simulink model "TRUAV_Dynamics_from_GTRS_trim"  (R2022b)
settings: Solver=ode4  StartTime=0.0  StopTime=3  FixedStep=0.004  RelTol=1e-3
values from neighbouring files (symbols this model uses):
  a_sound = 1116.45    [init_0_GTRS_data_Run_this_file.m]
  alpha_F_rad = alpha_F_deg * (pi/180)    [init_Vetical_2_Table.m]
  alpha_F_rad_table = alpha_F_table * (pi/180)    [init_Fuselage_Aero_Table.m]
  alpha_H_rad = alpha_H_deg * (pi/180)    [init_Horizontal_Table.m]
  alpha_HD_rad = alpha_HD_deg * (pi/180)    [init_Horizontal_C_D_Table.m]
  alpha_r0 = 0    [init_0_GTRS_data_Run_this_file.m]
  alpha_WF_epsilon_M_rad = alpha_WF_deg * pi/180    [init_WingWake_Deflection_Table.m]
  alpha_WS_CL_rad = alpha_WS_CL_deg * (pi/180)    [init_Wing_Slide_Table.m]
  b_w = 32.17    [init_0_GTRS_data_Run_this_file.m]
  beta_F_rad = beta_F_deg * (pi/180)    [init_Vetical_2_Table.m]
  beta_LD_rad_table = beta_LD_table * (pi/180)    [init_Fuselage_Aero_Table.m]
  beta_m_epsilon_M_rad = beta_m_deg * pi/180    [init_WingWake_Deflection_Table.m]
  beta_m_rad_cn = beta_m_deg_cn * pi/180    [init_Wing_Free_Table.m]
  beta_M_rad_table = beta_M_table  * (pi/180)    [init_Fuselage_Aero_Table.m]
  beta_m_S_rad = beta_m_S_deg * (pi/180)    [init_Vetical_2_Table.m]
  beta_m_WS_CL_rad = beta_m_WS_CL_deg * (pi/180)    [init_Wing_Slide_Table.m]
  beta_rad_brk = beta_KBR_rad    [init_Vetical_2_Table.m]
  beta_v_rad = beta_v_deg * (pi/180)    [init_Vetical_1_Table.m]
  beta_vD_rad = beta_vD_deg * (pi/180)    [init_Vetical_1_Table.m]
  beta_WF_Cl_rad = beta_W_deg * (pi/180)    [init_Wing_Free_Table.m]
  beta_WF_CL_rad = beta_CL_deg * (pi/180)    [init_Wing_Free_Table.m]
  beta_YlN_rad_table = beta_YlN_table * (pi/180)    [init_Fuselage_Aero_Table.m]
  c_HW = 3.92    [init_0_GTRS_data_Run_this_file.m]
  C_l_beta_CLwp_table = [ ... (first row only)    [init_Wing_Free_Table.m]
  C_l_beta_pro_CLwp_table = [ ... (first row only)    [init_Wing_Free_Table.m]
  C_L_delta_a_table = [0.00316, 0.00396, 0.00476, 0]    [init_Wing_Free_Table.m]
  C_LHB = -0.00422    [init_0_GTRS_data_Run_this_file.m]
  C_lp_C_LWP = -0.774    [init_0_GTRS_data_Run_this_file.m]
  C_m_wp_table = [ ... (first row only)    [init_Wing_Free_Table.m]
  C_MHA = 0    [init_0_GTRS_data_Run_this_file.m]
  C_MHO = 0    [init_0_GTRS_data_Run_this_file.m]
  c_R = 14/12    (= 1.16666666667)    [init_0_GTRS_data_Run_this_file.m]
  c_w = 5.225    [init_0_GTRS_data_Run_this_file.m]
  C_Y_beta = 0    [init_0_GTRS_data_Run_this_file.m]
  CD0_high_Mach_data = [0.0177, 0.0178, 0.0179, 0.0405]    [init_Wing_Free_Table.m]
  CD_4D_table = zeros(49, 4, 2, 4)    [init_Wing_Slide_Table.m]
  CDH_2D_table = zeros(length(alpha_HD_deg), length(mach_vec))    [init_Horizontal_C_D_Table.m]
  CDV_2D_table = zeros(length(beta_vD_deg), length(mach_vec))    [init_Vetical_1_Table.m]
  CL_4D_table = zeros(49, 4, 2, 4)    [init_Wing_Slide_Table.m]
  CLH_3D_table = zeros(length(alpha_H_deg), length(delta_e_deg), length(mach_vec))    [init_Horizontal_Table.m]
  CYV_3D_table = zeros(length(beta_v_deg), length(delta_r_deg), length(mach_vec))    [init_Vetical_1_Table.m]
  D_alpha_table = [D_part1, D_part2, D_part3, D_part4]    [init_Fuselage_Aero_Table.m]
  D_beta_table = [ fliplr(D_beta_half(2:end)),  D_beta_half]    [init_Fuselage_Aero_Table.m]
  D_ke = 0.24    [init_0_GTRS_data_Run_this_file.m]
  D_Kr = 0.24    [init_0_GTRS_data_Run_this_file.m]    (also in init_Vetical_1_Table.m)
  DBFO = -1.56    [init_0_GTRS_data_Run_this_file.m]
  delta_e_rad = delta_e_deg * (pi/180)    [init_Horizontal_Table.m]
  delta_r_deg = [-20, -15, 0, 15, 20]    [init_Vetical_1_Table.m]
  DLANG = -0.5    [init_0_GTRS_data_Run_this_file.m]
  epsilon_W_table = permute(epsilon_W_3D, [3, 1, 2])    [init_WingWake_Deflection_Table.m]
  flap_rad = flap_deg * (pi/180)    [init_Wing_Free_Table.m]    (also in init_Wing_Slide_Table.m)
  ft2m = 0.3048    [init_0_GTRS_data_Run_this_file.m]
  h_HW = [-0.5838, 0.01158, 0.5967, 0.002547,-2.2519]    [init_0_GTRS_data_Run_this_file.m]
  I_b = 102.5    [init_0_GTRS_data_Run_this_file.m]
  i_H = 0    [init_0_GTRS_data_Run_this_file.m]
  i_v = 0    [init_0_GTRS_data_Run_this_file.m]
  i_w = 0    [init_0_GTRS_data_Run_this_file.m]
  in2ft = 1/12    (= 0.0833333333333)    [init_0_GTRS_data_Run_this_file.m]
  Ixx = 52795    [init_0_GTRS_data_Run_this_file.m]
  Ixz = 1234    [init_0_GTRS_data_Run_this_file.m]
  Iyy = 21360    [init_0_GTRS_data_Run_this_file.m]
  Izz = 66335    [init_0_GTRS_data_Run_this_file.m]
  K1delta_data = [ ... (first row only)    [init_Wing_Free_Table.m]
  K_coeffs = [1.6 0]    [init_0_GTRS_data_Run_this_file.m]
  K_FWDF = -0.0035    [init_0_GTRS_data_Run_this_file.m]
  K_FWO = 1.4    [init_0_GTRS_data_Run_this_file.m]
  K_HNU = 0.8    [init_0_GTRS_data_Run_this_file.m]
  K_vNU = 1    [init_Vetical_1_Table.m]
  KBR_table = KBR_table_full    [init_Vetical_2_Table.m]
  Kn_delta_data = [ ... (first row only)    [init_Wing_Free_Table.m]
  Kno_delta_data = [ ... (first row only)    [init_Wing_Free_Table.m]
  L_alpha_table = [L_part1, L_part2, L_part3, L_part4]    [init_Fuselage_Aero_Table.m]
  L_beta_table = [ fliplr(L_beta_half(2:end)),  L_beta_half]    [init_Fuselage_Aero_Table.m]
  l_beta_table = [l_beta_neg, l_beta_pos]    [init_Fuselage_Aero_Table.m]
  L_n = 4.667    [init_0_GTRS_data_Run_this_file.m]
  lambda_w = -6.5*deg2rad    (= -0.11344640138)    [init_0_GTRS_data_Run_this_file.m]
  LBFO = -7.23    [init_0_GTRS_data_Run_this_file.m]
  LLANG = 0    [init_0_GTRS_data_Run_this_file.m]
  m2ft = 1/ft2m    (= 3.28083989501)    [init_0_GTRS_data_Run_this_file.m]
  M_alpha_table = [M_part1, M_part2, M_part3, M_part4]    [init_Fuselage_Aero_Table.m]
  M_beta_table = [ fliplr(M_beta_half(2:end)), M_beta_half]    [init_Fuselage_Aero_Table.m]
  Mach_brk = [0.2, 0.4, 0.5, 0.6]    [init_Wing_Free_Table.m]
  mach_vec = [0.2, 0.4, 0.5, 0.6]    [init_Horizontal_C_D_Table.m]    (also in init_Horizontal_Table.m; init_Vetical_1_Table.m)
  mass = 403.7    [init_0_GTRS_data_Run_this_file.m]
  mast_rad = mast_deg * pi/180    [init_Wing_Free_Table.m]
  MBFO = 66.5    [init_0_GTRS_data_Run_this_file.m]
  Mn_X_ke = [0 0.2 0.4 0.5 0.6 0.7]    [init_Horizontal_Table.m]
  N_beta_table = [N_beta_neg, N_beta_pos]    [init_Fuselage_Aero_Table.m]
  pos_x_CG = 300    [init_0_GTRS_data_Run_this_file.m]
  pos_x_H = 300    [init_0_GTRS_data_Run_this_file.m]
  pos_x_HW = 560    [init_0_GTRS_data_Run_this_file.m]
  pos_x_Nac = 291.7    [init_0_GTRS_data_Run_this_file.m]
  pos_x_V = 570    [init_0_GTRS_data_Run_this_file.m]
  pos_x_W = 291.7    [init_0_GTRS_data_Run_this_file.m]
  pos_y_CG = 0    [init_0_GTRS_data_Run_this_file.m]
  pos_y_H = 193    [init_0_GTRS_data_Run_this_file.m]
  pos_y_HW = 0    [init_0_GTRS_data_Run_this_file.m]
  pos_y_Nac = 193    [init_0_GTRS_data_Run_this_file.m]
  pos_y_V = 115.69    [init_0_GTRS_data_Run_this_file.m]
  pos_y_W = 96.6    [init_0_GTRS_data_Run_this_file.m]
  pos_z_CG = 81.65    [init_0_GTRS_data_Run_this_file.m]
  pos_z_H = 100    [init_0_GTRS_data_Run_this_file.m]
  pos_z_HW = 103    [init_0_GTRS_data_Run_this_file.m]
  pos_z_Nac = 118    [init_0_GTRS_data_Run_this_file.m]
  pos_z_V = 77    [init_0_GTRS_data_Run_this_file.m]
  pos_z_W = 96    [init_0_GTRS_data_Run_this_file.m]
  R = 12.5    [init_0_GTRS_data_Run_this_file.m]
  rho = 0.002376    [init_0_GTRS_data_Run_this_file.m]
  s_HW = 50.25    [init_0_GTRS_data_Run_this_file.m]
  S_max = 56    [init_0_GTRS_data_Run_this_file.m]
  S_v = 20.25    [init_0_GTRS_data_Run_this_file.m]
  S_w = 181    [init_0_GTRS_data_Run_this_file.m]
  Sidewash_4D = zeros(length(alpha_F_deg), length(beta_F_deg), length(beta_m_S_deg), length(delta_F_S_deg))    [init_Vetical_2_Table.m]
  slugft2kgm = 1.35582    [init_0_GTRS_data_Run_this_file.m]
  tau_e = 0.518    [init_0_GTRS_data_Run_this_file.m]
  tau_r = 0.27    [init_0_GTRS_data_Run_this_file.m]    (also in init_Vetical_1_Table.m)
  theta_0_R = 0.750    (= 0.75)    [init_0_GTRS_data_Run_this_file.m]
  theta_0_W = 1.187    [init_0_GTRS_data_Run_this_file.m]
  theta_twist = -41*deg2rad    (= -0.715584993318)    [init_0_GTRS_data_Run_this_file.m]
  u_max = 1181/12    (= 98.4166666667)    [init_0_GTRS_data_Run_this_file.m]
  ... (+3 more)
undefined symbols (not defined in the file or in its folder): beta_m_rad, F, Light, MIL, sigbuilder_block, tilt_cmd
libraries: simulink x2, sharedtransform x2, aerolibasang x2, aerolibwind2 x1
(part 4 of 4)

== matlab function TRUAV_Dynamics_from_GTRS_trim/Force and Moments/Propulsion1/Rotor Assembly 1 Right/叶素法 ==
  data: para input; AB input; V_H input; r_n input; beta_F_params input; Psi_1 input; v_i input; a_MR input; F_b output; M_b output; delta_H input; T_NAC2B input; T_H2NAC input; beta_F output; Thrust_mag output
function [F_b, M_b, beta_F, Thrust_mag] = F_M_rotor(para,AB, V_H, r_n, beta_F_params, Psi_1, ...
                                           v_i, a_MR, delta_H, T_NAC2B, T_H2NAC)
% =========================================================================
% 全旋翼（3叶片）叶素积分气动力与力矩计算函数
% =========================================================================

    % ========== 0. 参数读取 =============
    R = para(1);
    theta_twist = para(2); % 扭转率
    rho = para(3);
    c_R = para(4);a_sound = para(5);

    Nb = 3;                % 桨叶数 (XV-15/V-22均为3叶)
    
    theta_all = AB(1);     % 总距
    A1 = AB(2); B1 = AB(3); % 横向、纵向周期变距
    
    % 从第二段代码传入的挥舞傅里叶系数
    a0  = beta_F_params(1);
    a1s = beta_F_params(2);
    b1s = beta_F_params(3);

    delta_H = delta_H(:); % 无论输入是什么形状，强行拉直为列向量
    
    N_segments = 40;
    dr = R / N_segments;
    r_vec = (0.5:1:N_segments-0.5)' * dr; 
    x = r_vec / R;
    
    % 初始化整个旋翼在桨毂系(Hub)下的总力和总力矩
    % 初始化整个旋翼在桨毂系(Hub)下的总力和总力矩
    F_HUB_total = zeros(3,1); 
    M_HUB_total = zeros(3,1); 
    
    % ========== 改造点：方位角离散平均法 ==========
    N_azimuth = 36; % 将一圈分为 36 份 (每 10 度算一次)
    dPsi = 2 * pi / N_azimuth;
    
    for k = 1:N_azimuth
        % 虚拟桨叶当前的方位角
        Psi = (k - 1) * dPsi; 
        
        % 根据傅里叶级数实时计算该方位角下的挥舞角和角速度
        beta_F = a0 - a1s*cos(Psi) - b1s*sin(Psi);
        beta_dot = r_n * (a1s*sin(Psi) - b1s*cos(Psi));
        
        dY_prime = zeros(N_segments, 1);
        dZ_prime = zeros(N_segments, 1);
        dQ_torque = zeros(N_segments, 1);
        
        % ========== 2. 逐段计算叶素气动力 ==========
        for i = 1:N_segments
            r_local = r_vec(i);
            
            % 【修复提醒】：请用回正确的面内速度矢量分解！
            % (不要用 sqrt 标量化，否则侧飞时力矩会错)
            U_T = r_n * r_local + V_H(1) * sin(Psi) - V_H(2) * cos(Psi); 
            U_R = V_H(1) * cos(Psi) + V_H(2) * sin(Psi);
            U_P = r_local * beta_dot + U_R * beta_F + V_H(3) + v_i;
            
            if U_T < 0; U_T = abs(U_T); end
            
            phi_b = atan2(U_P, U_T);
            theta = theta_all + A1*cos(Psi) + B1*sin(Psi) + theta_twist*x(i);
            alpha_blade = theta - phi_b;
            
            U = sqrt(U_T^2 + U_P^2);
            M_local = U / a_sound;
            abs_alpha = abs(alpha_blade);
            cd_base = 0.015 + abs_alpha * (0.068 + abs_alpha * 0.81);
            comp_term = 0.01 * abs_alpha + 0.02 *(0.85+ max(M_local,0.35)); 
            cd_comp = max(0, comp_term);
            cd_local = min(0.11, cd_base + cd_comp);
            
            dL = 0.5 * rho * U^2 * a_MR * alpha_blade * c_R * dr;
            dD = 0.5 * rho * U^2 * cd_local * c_R * dr;
            
            dY_prime(i) = dL * sin(phi_b) + dD * cos(phi_b);
            dZ_prime(i) = dL * cos(phi_b) - dD * sin(phi_b);
            dQ_torque(i) = dY_prime(i) * r_local; 
        end
        
        Y_prime = sum(dY_prime);   
        Z_prime = sum(dZ_prime);   
        Q_blade = sum(dQ_torque);  
        F_blade_local = [0; Y_prime; Z_prime]; 
        
        % 3.1 挥舞矩阵 (绕 Y 轴向上翘起 beta)
        % 注意：因为桨叶沿 X 轴伸出，挥舞必须绕 Y 轴！
        T_Flap2Rot = [ cos(beta_F),  0, -sin(beta_F);
                                 0,  1,           0;
                       sin(beta_F),  0,  cos(beta_F)];
        % 旋转系到桨毂系
        T_R2H = [cos(Psi), -sin(Psi),  0;
                 sin(Psi),  cos(Psi),  0;
                        0,         0,  1];
                     
        F_HUB_blade = T_R2H * T_Flap2Rot * F_blade_local;
        
        % 累加这个方位角切片上的力
        F_HUB_total = F_HUB_total + F_HUB_blade;
        M_HUB_total(3) = M_HUB_total(3) + Q_blade; 
    end
    
    % ========== 3. 求一圈的平均力，再乘以真实桨叶数 ==========
    % 因为我们积了 36 次，相当于有 36 片桨叶，所以要除以 36，再乘以真实的 3 片
    F_HUB_total = F_HUB_total * (Nb / N_azimuth);
    M_HUB_total = M_HUB_total * (Nb / N_azimuth);
    
    % ... 下面的 T_HUB2BODY 和 cross(delta_H, F_b) 保持不变 ...
    % ========== 4. 转换到机体轴系 (Body Frame) ==========
    % 矩阵相乘顺序：F_body = T(Nac->Body) * T(Hub->Nac) * F_hub
    % 注意检查 T_H2NAC 等矩阵的定义，确保是 "坐标系变换矩阵" 还是 "向量变换矩阵"
    
    T_HUB2BODY = T_NAC2B * T_H2NAC; 
    
    F_b = T_HUB2BODY * F_HUB_total;

    Thrust_mag = abs(F_HUB_total(3));
    
    % 桨毂自身的力矩（扭矩）也要转到机体系
    M_hub_body = T_HUB2BODY * M_HUB_total;
    
    % ========== 5. 计算最终重心的总力矩 ==========
    % 总力矩 = 旋翼产生的基础力矩 + 重心力臂产生的附加力矩
    M_b = M_hub_body + cross(delta_H, F_b);
%       M_b = M_hub_body ;

end

== matlab function TRUAV_Dynamics_from_GTRS_trim/Force and Moments/Propulsion1/Rotor Assembly 1 Right/旋转矩阵计算 ==
  data: T_H2NAC output; tilt input; T_NAC2B output
function [T_H2NAC ,T_NAC2B]  = Transf(tilt)

T_H2NAC = [-1     0     0;
          0     1     0;
          0     0     -1];

T_NAC2B = [cos(tilt)  0     -sin(tilt);
           0          1       0;
           sin(tilt)  0     cos(tilt)];

== matlab function TRUAV_Dynamics_from_GTRS_trim/Force and Moments/Propulsion1/Rotor Assembly 1 Right/桨毂中心速度、前进比、 侧滑角、入流比、诱导速度 ==
  data: Para input; V_H output; tilt input; CG input; CT input; mu output; beta_w output; omega input; r_n input; V_body input; T_H2NAC input; lamda output; v_i output; POS_H output; T_NAC2B input
function [V_H, mu, beta_w, lamda, v_i, POS_H] = fcn(Para, tilt, CG, CT, omega, r_n, V_body, T_H2NAC, T_NAC2B)

    % ========== 解析结构参数 ==========
    SL_SP = Para(1);     % 枢轴点纵向位置 [in]
    BL_SP = Para(2);     % 枢轴点横向位置 [in]
    WL_SP = Para(3);     % 枢轴点垂向位置 [in]
    L_n = Para(4);  
    R = Para(5);
    
    Omega_R = r_n * R;   % 预计算桨尖速度

   % ========== 计算桨毂中心绝对位置 (NASA 体系) ==========
    % x_H 公式没问题：倾转 90 度时，桨毂向前伸出 L_n，FS 变小
    x_H = SL_SP - L_n * sin(tilt); 
    
    y_H = BL_SP; 
    
    % z_H 必须修正：直升机模式 (tilt=0) 时最高，固定翼模式 (tilt=90) 时放平
    z_H = WL_SP + L_n * cos(tilt);

    % ========== 计算重心与桨毂中心相对位置 ==========
    x_BH = CG(1) - x_H;
    y_BH = -CG(2) + y_H;                  % [in]
    z_BH = CG(3) - z_H;                  % [in]

    POS_H = [x_BH;y_BH;z_BH];

    % ========== 计算桨毂中心速度（桨毂系） ==========
%     Omega_skew = [ 0,         omega(3),  -omega(2);
%                   -omega(3),  0,          omega(1);
%                    omega(2), -omega(1),   0 ];
               
    % 先求出机体坐标系下的桨毂速度，再用转换矩阵转到桨毂系
%     V_H = T_H2NAC' * T_NAC2B' * (V_body + Omega_skew * [x_BH; y_BH; z_BH]);
     V_H = T_H2NAC' * T_NAC2B' * (V_body );

    % ========== 计算前进比和旋翼侧滑角 ==========
    % 注意：如果处于纯悬停，V_H(1)和V_H(2)为0，计算beta_w时需防止分母为0
    V_xy = sqrt(V_H(1)^2 + V_H(2)^2);
    mu = V_xy / Omega_R;
    
    if V_xy < 1e-5
        beta_w = 0; % 悬停时无明显侧滑角
    else
        beta_w = asin(V_H(2) / V_xy);
    end

    % ========== 调用独立的迭代函数求解入流比和诱导速度 ==========
    V_z = V_H(3);
    [lamda, v_i] = calc_rotor_inflow(mu, V_z, Omega_R, CT);

end
